simulink model "LPFSimulation"  (R2020a)
settings: Solver=VariableStepAuto  StartTime=0.0  StopTime=0.005  RelTol=1e-3
settings Model: Creator=victo  LastModifiedBy=lsjsa

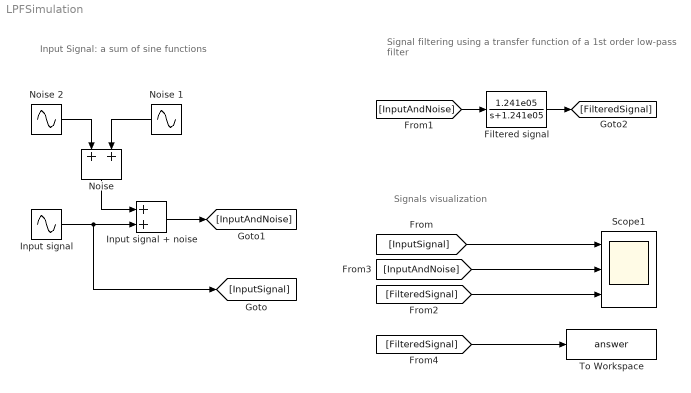
== system LPFSimulation ==
  note: Signals visualization
  note: Signal filtering using a transfer function of a 1st order low-pass filter
  note: Input Signal: a sum of sine functions
  Filtered signal : TransferFcn  Numerator=[0, 1.241e05]  Denominator=[1, 1.241e05]
  Input signal : Sin  Frequency=2000*pi  SampleTime=0
  Input signal + noise : Sum
  Noise : Sum
  Noise 1 : Sin  Frequency=80000*pi  SampleTime=0
  Noise 2 : Sin  Frequency=50000*pi  SampleTime=0
  Scope1 : Scope  NumInputPorts=3
  To Workspace : ToWorkspace  VariableName=answer  SaveFormat=Timeseries  SampleTime=-1
  wires:
  Input signal/1 -> [InputSignal], Input signal + noise/2
  Noise 1/1 -> Noise/2
  Noise/1 -> Input signal + noise/1
  Noise 2/1 -> Noise/1
  [InputSignal] -> Scope1/1
  Input signal + noise/1 -> [InputAndNoise]
  [InputAndNoise] -> Filtered signal/1
  Filtered signal/1 -> [FilteredSignal]
  [FilteredSignal] -> Scope1/3
  [InputAndNoise] -> Scope1/2
  [FilteredSignal] -> To Workspace/1
